simulink model "TPS_SensorV20"  (R2020a)
settings: Solver=FixedStepDiscrete  StartTime=0.0  StopTime=10.0  FixedStep=.1  RelTol=1e-3
settings Model: Creator=Administrator  LastModifiedBy=Administrator
settings OptimizationCC: DefaultParameterBehavior=Inlined  EnhancedBackFolding=on  PassReuseOutputArgsAs=Individual arguments  ZeroExternalMemoryAtStartup=off  ZeroInternalMemoryAtStartup=off  OptimizeBlockOrder=speed  DifferentSizesBufferReuse=on  OptimizationCustomize=off  EfficientTunableParamExpr=on
settings DebuggingCC: ParameterTunabilityLossMsg=error  UnconnectedInputMsg=none  UnconnectedOutputMsg=none  UnconnectedLineMsg=none
settings HardwareCC: ProdBitPerPointer=32  ProdBitPerSizeT=32  ProdBitPerPtrDiffT=32  ProdLargestAtomicInteger=Long  ProdLargestAtomicFloat=Double  ProdWordSize=32  ProdHWDeviceType=ARM Compatible->ARM Cortex
settings ModelReferenceCC: EnableRefExpFcnMdlSchedulingChecks=off
settings SFSimCC: MATLABDynamicMemAlloc=off
settings RTWCC: SystemTargetFile=ert.tlc  GenCodeOnly=on  TemplateMakefile=ert_default_tmf
settings CodeAppCC: ForceParamTrailComments=on  IgnoreCustomStorageClasses=off  OperatorAnnotations=on  SimulinkDataObjDesc=on  SFDataObjDesc=on  InsertBlockDesc=on
settings ERTTargetCC: TargetLangStandard=C99 (ISO)  GenerateSampleERTMain=on  InlinedParameterPlacement=NonHierarchical  ERTCustomFileTemplate=example_file_process.tlc

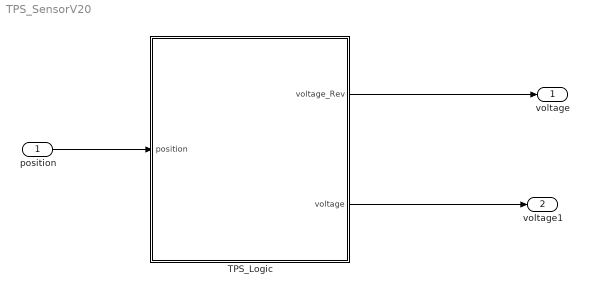
== system TPS_SensorV20 ==
  position : Inport
  TPS_Logic : Subsystem  TreatAsAtomicUnit=on
  voltage : Outport
  voltage1 : Outport  Port=2
  wires:
  TPS_Logic/1(voltage_Rev) -> voltage/1
  TPS_Logic/2(voltage) -> voltage1/1
  position/1 -> TPS_Logic/1(position)

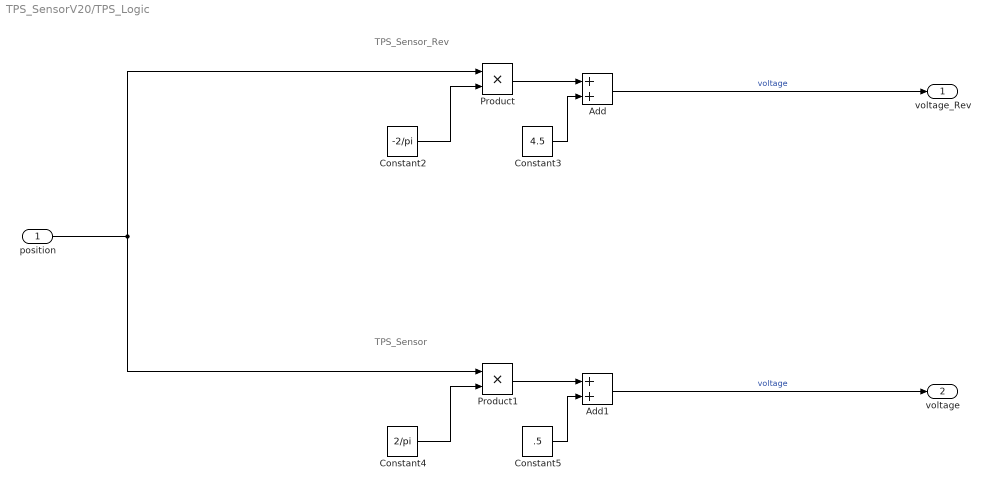
== system TPS_SensorV20/TPS_Logic ==
  note: TPS_Sensor
  note: TPS_Sensor_Rev
  position : Inport
  Add : Sum
  Add1 : Sum
  Constant2 : Constant  Value=-2/pi
  Constant3 : Constant  Value=4.5
  Constant4 : Constant  Value=2/pi
  Constant5 : Constant  Value=.5
  Product : Product
  Product1 : Product
  voltage_Rev : Outport
  voltage : Outport  Port=2
  wires:
  Product/1 -> Add/1
  Constant5/1 -> Add1/2
  Add1/1 -> voltage/1  "voltage"
  position/1 -> Product/1, Product1/1
  Constant4/1 -> Product1/2
  Constant2/1 -> Product/2
  Product1/1 -> Add1/1
  Constant3/1 -> Add/2
  Add/1 -> voltage_Rev/1  "voltage"
